simulink model "Case2simulimk"  (R2022b)
settings: Solver=FixedStepAuto  StartTime=0.0  StopTime=5  FixedStep=1e-4  RelTol=1e-3  EnableMultiTasking=on
undefined symbols (not defined in the file): Kb, Kb2, P, perd, rho, x0
settings Model: Creator=sf  LastModifiedBy=sf
settings ModelReferenceCC: EnableRefExpFcnMdlSchedulingChecks=on

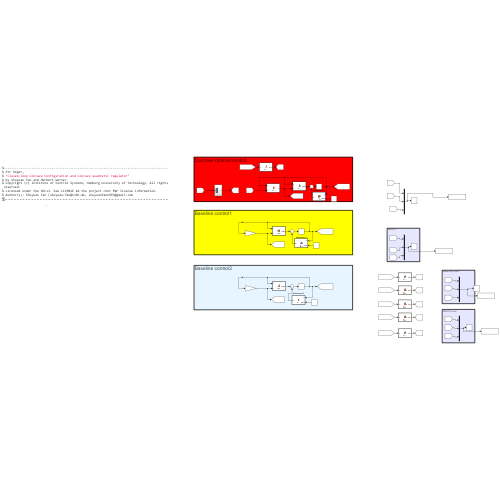
[thumbnail: Simulink's stored preview of the top-level diagram]
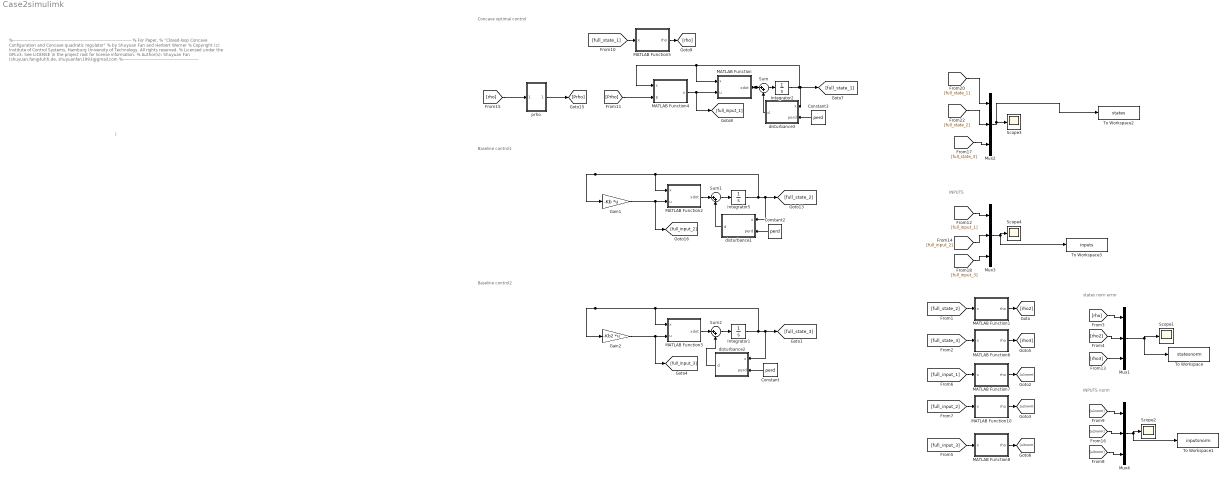
== system Case2simulimk ==
  note: )
  note: %-----------------------------------------------------------------------------------------
      | % For Paper,
      | % "Closed-loop Concave Configuration and Concave quadratic regulator"
      | % by Shuyuan Fan and Herbert Werner
      | % Copyright (c) Institute of Control Systems, Hamburg University of Technology. All rights reserved.
      | % Licensed under the GPLv3. See LICENSE in the project root for license information.
      | % Author(s): Shuyuan Fan (shuyuan.fan@tuhh.de, shuyuanfan1993@gmail.com
      | %---------------------------------------------------------
  note: INPUTS
  note: Baseline control1
  note: Concave optimal control
  note: states norn error
  note: INPUTS norm
  note: Baseline control2
  Constant : Constant  Value=perd
  Constant2 : Constant  Value=perd
  Constant3 : Constant  Value=perd
  Gain1 : Gain  Gain=-Kb  Multiplication=Matrix(K*u)
  Gain2 : Gain  Gain=-Kb2  Multiplication=Matrix(K*u)
  Integrator1 : Integrator  InitialCondition=x0
  Integrator2 : Integrator  InitialCondition=x0
  Integrator5 : Integrator  InitialCondition=x0
  MATLAB Function : MATLAB Function  TreatAsAtomicUnit=on
  MATLAB Function1 : MATLAB Function  TreatAsAtomicUnit=on
  MATLAB Function10 : MATLAB Function  TreatAsAtomicUnit=on
  MATLAB Function2 : MATLAB Function  TreatAsAtomicUnit=on
  MATLAB Function3 : MATLAB Function  TreatAsAtomicUnit=on
  MATLAB Function4 : MATLAB Function  TreatAsAtomicUnit=on
  MATLAB Function5 : MATLAB Function  TreatAsAtomicUnit=on
  MATLAB Function6 : MATLAB Function  TreatAsAtomicUnit=on
  MATLAB Function7 : MATLAB Function  TreatAsAtomicUnit=on
  MATLAB Function8 : MATLAB Function  TreatAsAtomicUnit=on
  Mux{1..4} (4 alike) : Mux  Inputs=3
  Scope{1..4} (4 alike) : Scope
  Sum : Sum  Inputs=|++
  Sum1 : Sum  Inputs=|++
  Sum2 : Sum  Inputs=|++
  To Workspace : ToWorkspace  VariableName=statesnorm  SaveFormat=Timeseries  SampleTime=-1
  To Workspace1 : ToWorkspace  VariableName=inputsnorm  SaveFormat=Timeseries  SampleTime=-1
  To Workspace2 : ToWorkspace  VariableName=states  SaveFormat=Timeseries  SampleTime=-1
  To Workspace3 : ToWorkspace  VariableName=inputs  SaveFormat=Timeseries  SampleTime=-1
  disturbance1 : MATLAB Function  TreatAsAtomicUnit=on
  disturbance2 : MATLAB Function  TreatAsAtomicUnit=on
  disturbance3 : MATLAB Function  TreatAsAtomicUnit=on
  prho : Subsystem
  wires:
  Mux3/1 -> Scope4/1, To Workspace3/1
  MATLAB Function5/1(rho) -> [rho]
  [full_state_1] -> Mux2/1
  MATLAB Function2/1(xdot) -> Sum1/1
  [full_state_2] -> Mux2/2
  Gain1/1 -> MATLAB Function2/2(u), [full_input_2]
  Mux2/1 -> Scope3/1, To Workspace2/1
  [rho] -> prho/1(In1)
  prho/1(Out1) -> [Prho]
  [full_input_1] -> Mux3/1
  [full_input_2] -> Mux3/2
  [full_state_1] -> MATLAB Function5/1(x)
  MATLAB Function4/1(u) -> MATLAB Function/2(u), [full_input_1]
  MATLAB Function/1(xdot) -> Sum/1
  [Prho] -> MATLAB Function4/2(p)
  [full_state_2] -> MATLAB Function1/1(x)
  [full_input_2] -> MATLAB Function10/1(x)
  MATLAB Function7/1(rho) -> [u1norm]
  MATLAB Function1/1(rho) -> [rho2]
  MATLAB Function10/1(rho) -> [u2norm]
  [full_input_1] -> MATLAB Function7/1(x)
  [u2norm] -> Mux4/2
  [rho] -> Mux1/1
  [rho2] -> Mux1/2
  Mux4/1 -> Scope2/1, To Workspace1/1
  Mux1/1 -> Scope1/1, To Workspace/1
  [u1norm] -> Mux4/1
  Integrator2/1 -> MATLAB Function4/1(x), MATLAB Function/1(x), disturbance3/1(x), [full_state_1]
  Integrator5/1 -> disturbance1/1(x), [full_state_2], Gain1/1, MATLAB Function2/1(x)
  Integrator1/1 -> disturbance2/1(x), [full_state_3], Gain2/1, MATLAB Function3/1(x)
  Gain2/1 -> MATLAB Function3/2(u), [full_input_3]
  MATLAB Function3/1(xdot) -> Sum2/1
  MATLAB Function6/1(rho) -> [rho3]
  [full_state_3] -> MATLAB Function6/1(x)
  [full_input_3] -> MATLAB Function8/1(x)
  MATLAB Function8/1(rho) -> [u3norm]
  [u3norm] -> Mux4/3
  [rho3] -> Mux1/3
  [full_state_3] -> Mux2/3
  [full_input_3] -> Mux3/3
  Sum/1 -> Integrator2/1
  Sum1/1 -> Integrator5/1
  Sum2/1 -> Integrator1/1
  disturbance2/1(d) -> Sum2/2
  Constant/1 -> disturbance2/2(perd)
  Constant2/1 -> disturbance1/2(perd)
  disturbance1/1(d) -> Sum1/2
  Constant3/1 -> disturbance3/2(perd)
  disturbance3/1(d) -> Sum/2

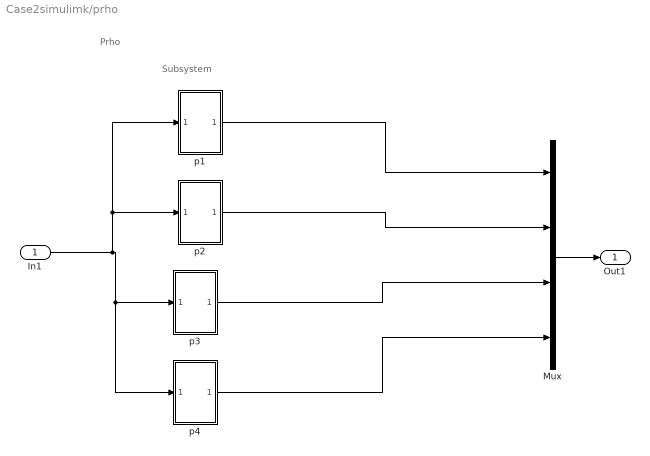
== system Case2simulimk/prho ==
  note: Prho
  note: Subsystem
  In1 : Inport
  Mux : Mux
  p1 : Subsystem
  p2 : Subsystem
  p3 : Subsystem
  p4 : Subsystem
  Out1 : Outport
  wires:
  p4/1(Out1) -> Mux/4
  In1/1 -> p4/1(In1), p3/1(In1), p2/1(In1), p1/1(In1)
  Mux/1 -> Out1/1
  p1/1(Out1) -> Mux/1
  p3/1(Out1) -> Mux/3
  p2/1(Out1) -> Mux/2

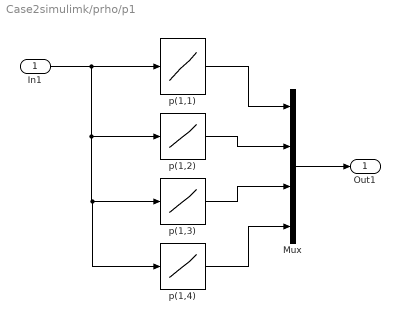
== system Case2simulimk/prho/p1 ==
  In1 : Inport
  Mux : Mux
  p(1,1) : Lookup_n-D  NumberOfTableDimensions=1  BreakpointsForDimension1=rho  Table=P(:,1)  InterpMethod=Linear Lagrange  InternalRulePriority=Speed  RndMeth=Simplest
  p(1,2) : Lookup_n-D  NumberOfTableDimensions=1  BreakpointsForDimension1=rho  Table=P(:,2)  InterpMethod=Linear Lagrange  InternalRulePriority=Speed  RndMeth=Simplest
  p(1,3) : Lookup_n-D  NumberOfTableDimensions=1  BreakpointsForDimension1=rho  Table=P(:,2)  InterpMethod=Linear Lagrange  InternalRulePriority=Speed  RndMeth=Simplest
  p(1,4) : Lookup_n-D  NumberOfTableDimensions=1  BreakpointsForDimension1=rho  Table=P(:,4)  InterpMethod=Linear Lagrange  InternalRulePriority=Speed  RndMeth=Simplest
  Out1 : Outport
  wires:
  p(1,2)/1 -> Mux/2
  p(1,4)/1 -> Mux/4
  In1/1 -> p(1,4)/1, p(1,3)/1, p(1,2)/1, p(1,1)/1
  p(1,1)/1 -> Mux/1
  p(1,3)/1 -> Mux/3
  Mux/1 -> Out1/1

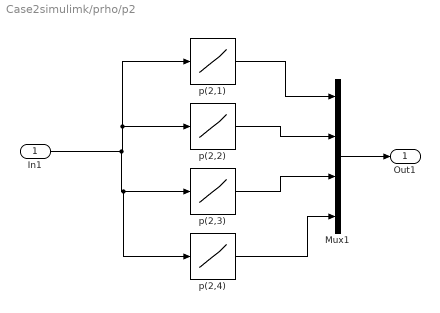
== system Case2simulimk/prho/p2 ==
  In1 : Inport
  Mux1 : Mux
  p(2,1) : Lookup_n-D  NumberOfTableDimensions=1  BreakpointsForDimension1=rho  Table=P(:,5)  InterpMethod=Linear Lagrange  InternalRulePriority=Speed  RndMeth=Simplest
  p(2,2) : Lookup_n-D  NumberOfTableDimensions=1  BreakpointsForDimension1=rho  Table=P(:,6)  InterpMethod=Linear Lagrange  InternalRulePriority=Speed  RndMeth=Simplest
  p(2,3) : Lookup_n-D  NumberOfTableDimensions=1  BreakpointsForDimension1=rho  Table=P(:,7)  InterpMethod=Linear Lagrange  InternalRulePriority=Speed  RndMeth=Simplest
  p(2,4) : Lookup_n-D  NumberOfTableDimensions=1  BreakpointsForDimension1=rho  Table=P(:,8)  InterpMethod=Linear Lagrange  InternalRulePriority=Speed  RndMeth=Simplest
  Out1 : Outport
  wires:
  In1/1 -> p(2,4)/1, p(2,3)/1, p(2,2)/1, p(2,1)/1
  Mux1/1 -> Out1/1
  p(2,4)/1 -> Mux1/4
  p(2,2)/1 -> Mux1/2
  p(2,3)/1 -> Mux1/3
  p(2,1)/1 -> Mux1/1

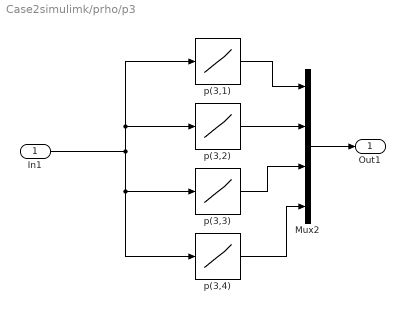
== system Case2simulimk/prho/p3 ==
  In1 : Inport
  Mux2 : Mux
  p(3,1) : Lookup_n-D  NumberOfTableDimensions=1  BreakpointsForDimension1=rho  Table=P(:,9)  InterpMethod=Linear Lagrange  InternalRulePriority=Speed  RndMeth=Simplest
  p(3,2) : Lookup_n-D  NumberOfTableDimensions=1  BreakpointsForDimension1=rho  Table=P(:,10)  InterpMethod=Linear Lagrange  InternalRulePriority=Speed  RndMeth=Simplest
  p(3,3) : Lookup_n-D  NumberOfTableDimensions=1  BreakpointsForDimension1=rho  Table=P(:,11)  InterpMethod=Linear Lagrange  InternalRulePriority=Speed  RndMeth=Simplest
  p(3,4) : Lookup_n-D  NumberOfTableDimensions=1  BreakpointsForDimension1=rho  Table=P(:,12)  InterpMethod=Linear Lagrange  InternalRulePriority=Speed  RndMeth=Simplest
  Out1 : Outport
  wires:
  p(3,4)/1 -> Mux2/4
  In1/1 -> p(3,4)/1, p(3,3)/1, p(3,2)/1, p(3,1)/1
  p(3,1)/1 -> Mux2/1
  p(3,2)/1 -> Mux2/2
  p(3,3)/1 -> Mux2/3
  Mux2/1 -> Out1/1

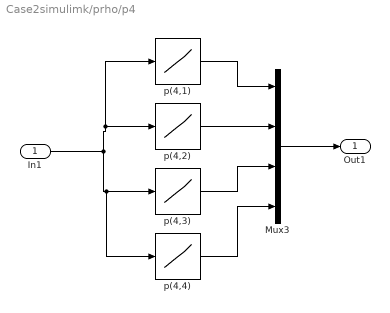
== system Case2simulimk/prho/p4 ==
  In1 : Inport
  Mux3 : Mux
  p(4,1) : Lookup_n-D  NumberOfTableDimensions=1  BreakpointsForDimension1=rho  Table=P(:,13)  InterpMethod=Linear Lagrange  InternalRulePriority=Speed  RndMeth=Simplest
  p(4,2) : Lookup_n-D  NumberOfTableDimensions=1  BreakpointsForDimension1=rho  Table=P(:,14)  InterpMethod=Linear Lagrange  InternalRulePriority=Speed  RndMeth=Simplest
  p(4,3) : Lookup_n-D  NumberOfTableDimensions=1  BreakpointsForDimension1=rho  Table=P(:,15)  InterpMethod=Linear Lagrange  InternalRulePriority=Speed  RndMeth=Simplest
  p(4,4) : Lookup_n-D  NumberOfTableDimensions=1  BreakpointsForDimension1=rho  Table=P(:,16)  InterpMethod=Linear Lagrange  InternalRulePriority=Speed  RndMeth=Simplest
  Out1 : Outport
  wires:
  p(4,2)/1 -> Mux3/2
  p(4,3)/1 -> Mux3/3
  In1/1 -> p(4,2)/1, p(4,1)/1, p(4,4)/1, p(4,3)/1
  Mux3/1 -> Out1/1
  p(4,1)/1 -> Mux3/1
  p(4,4)/1 -> Mux3/4

== matlab function Case2simulimk/MATLAB Function ==
  data: x input; u input; xdot output
function xdot = fcn(x,u)
%% model from paper "Design and Flight testing evaluation of formation control laws (2006)"
% https://ieeexplore.ieee.org/stamp/stamp.jsp?tp=&arnumber=1709935
% state space model

A = [0.430   0.094   -1.030   0.237;...
    -67.334  -7.949   5.640      0;...
    20.533    -0.655  -1.996    0;...
       0        1        0       0];

B = [0.272  -0.771;...
     -101.845  33.474;...
     -6.261   -24.363;...
       0     0];

xdot = A*x + B*u;

end

== matlab function Case2simulimk/MATLAB Function2 ==
  data: x input; u input; xdot output
function xdot = fcn(x,u)
%% model from paper "Design and Flight testing evaluation of formation control laws (2006)"
% https://ieeexplore.ieee.org/stamp/stamp.jsp?tp=&arnumber=1709935
% state space model

A = [0.430   0.094   -1.030   0.237;...
    -67.334  -7.949   5.640      0;...
    20.533    -0.655  -1.996    0;...
       0        1        0       0];

B = [0.272  -0.771;...
     -101.845  33.474;...
     -6.261   -24.363;...
       0     0];

xdot = A*x + B*u;

end

== matlab function Case2simulimk/MATLAB Function10 ==
  data: x input; rho output
function rho = fcn(x)

rho = sqrt(x'*x);

== matlab function Case2simulimk/MATLAB Function3 ==
  data: x input; u input; xdot output
function xdot = fcn(x,u)
%% model from paper "Design and Flight testing evaluation of formation control laws (2006)"
% https://ieeexplore.ieee.org/stamp/stamp.jsp?tp=&arnumber=1709935
% state space model

A = [0.430   0.094   -1.030   0.237;...
    -67.334  -7.949   5.640      0;...
    20.533    -0.655  -1.996    0;...
       0        1        0       0];

B = [0.272  -0.771;...
     -101.845  33.474;...
     -6.261   -24.363;...
       0     0];

xdot = A*x + B*u;

end

== matlab function Case2simulimk/MATLAB Function4 ==
  data: x input; u output; p input
function u= fcn(x,p)
R = diag([1,1]);
% system matrix
A = [0.430   0.094   -1.030   0.237;...
    -67.334  -7.949   5.640      0;...
    20.533    -0.655  -1.996    0;...
       0        1        0       0];

B = [0.272  -0.771;...
     -101.845  33.474;...
     -6.261   -24.363;...
       0     0];
p_ = reshape(p,[4,4]);
P = p_';
R_inv = inv(R);
u = -R_inv*B'*P*x;

== matlab function Case2simulimk/MATLAB Function7 ==
  data: x input; rho output
function rho = fcn(x)

rho = sqrt(x'*x);

== matlab function Case2simulimk/MATLAB Function6 ==
  data: x input; rho output
function rho = fcn(x)

rho = sqrt(x'*x);

== matlab function Case2simulimk/MATLAB Function8 ==
  data: x input; rho output
function rho = fcn(x)

rho = sqrt(x'*x);

== matlab function Case2simulimk/MATLAB Function5 ==
  data: x input; rho output
function rho = fcn(x)

rho = sqrt(x'*x);

== matlab function Case2simulimk/MATLAB Function1 ==
  data: x input; rho output
function rho = fcn(x)

rho = sqrt(x'*x);

== matlab function Case2simulimk/disturbance2 ==
  data: x input; d output; perd input
function d = fcn(x,perd)

d1 = 0;
d2 =0;
d3 =0;
d4 = 1*sin(10*x(4));

d = perd * [d1;d2;d3;d4];

== matlab function Case2simulimk/disturbance1 ==
  data: x input; d output; perd input
function d = fcn(x,perd)

d1 = 0;
d2 =0;
d3 =0;
d4 = 1*sin(10*x(4));

d = perd * [d1;d2;d3;d4];

== matlab function Case2simulimk/disturbance3 ==
  data: x input; d output; perd input
function d = fcn(x,perd)

d1 = 0;
d2 =0;
d3 =0;
d4 = 1*sin(10*x(4));

d = perd * [d1;d2;d3;d4];
